simulink model "Eq6_StorageLoss"  (R2022b)
settings: Solver=FixedStepAuto  StartTime=0.0  StopTime=10.0  RelTol=1e-3
settings Model: Creator=umber  LastModifiedBy=umber
settings OptimizationCC: OptimizeBlockIOStorage=off  OptimizeDataStoreBuffers=off  BusAssignmentInplaceUpdate=off
settings DebuggingCC: SFUnexpectedBacktrackingDiag=warning  SFNoUnconditionalDefaultTransitionDiag=warning
settings ModelReferenceCC: EnableRefExpFcnMdlSchedulingChecks=on
settings RTWCC: GenerateReport=on  BuildConfiguration=Debug  LaunchReport=on
settings CodeAppCC: ForceParamTrailComments=on  MATLABSourceComments=on  EnableCustomComments=on
settings GRTTargetCC: CombineSignalStateStructs=on  SupportVariableSizeSignals=on  MultiInstanceErrorCode=Warning

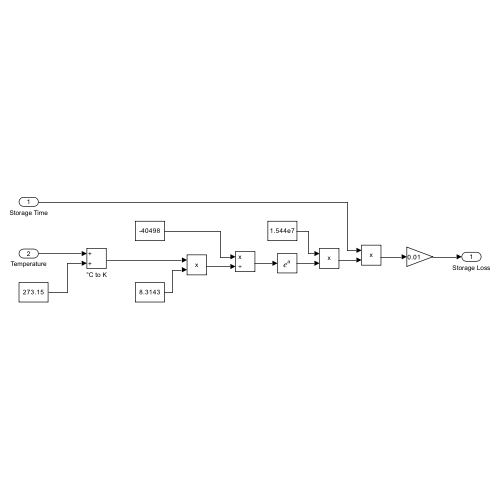
[thumbnail: Simulink's stored preview of the top-level diagram]
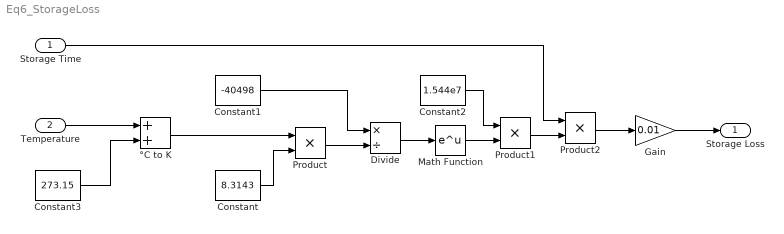
== system Eq6_StorageLoss ==
  Storage Time : Inport
  Temperature : Inport  Port=2
  Constant : Constant  Value=8.3143
  Constant1 : Constant  Value=-40498
  Constant2 : Constant  Value=1.544e7
  Constant3 : Constant  Value=273.15
  Divide : Product  Inputs=*/
  Gain : Gain  Gain=0.01
  Math Function : Math
  Product : Product
  Product1 : Product
  Product2 : Product
  °C to K : Sum
  Storage Loss : Outport
  wires:
  Constant/1 -> Product/2
  Temperature/1 -> °C to K/1
  Product/1 -> Divide/2
  Constant1/1 -> Divide/1
  Divide/1 -> Math Function/1
  Math Function/1 -> Product1/2
  Constant2/1 -> Product1/1
  Product1/1 -> Product2/2
  Storage Time/1 -> Product2/1
  Product2/1 -> Gain/1
  Gain/1 -> Storage Loss/1
  °C to K/1 -> Product/1
  Constant3/1 -> °C to K/2
